simulink model "Feuchtesimulation_G21_EU6AGA_rueckgabewerte"  (R2021b)
settings: Solver=FixedStepAuto  StartTime=start_time  StopTime=stop_time  FixedStep=ts  RelTol=1e-3
undefined symbols (not defined in the file or in its folder): A_Kat0, A_Kat1, A_Kat2, A_Kat3, A_Mantel_Kat0, A_Mantel_Kat1, A_Mantel_Kat2, A_Mantel_Kat3, Air_N2, Air_O2, beladungskennfeld, C_mw, CO2_mw, FeuchteAnsaugluft_rel, FeuchtegradAnsaugluft, Fuel_C, Fuel_H, H2O_mw, H_mw, Kat0_Anzahl_Zonen, Kat1_Anzahl_Zonen, Kat2_Anzahl_Zonen, Kat3_Anzahl_Zonen, l_Kat0, l_Kat1, l_Kat2, l_Kat3, m_Canning_Kat0, m_Canning_Kat1, m_Canning_Kat2, m_Canning_Kat3, m_h2o_kat0_ads, m_h2o_kat0_kond, m_h2o_kat1_ads, m_h2o_kat1_kond, m_h2o_kat2_ads, m_h2o_kat2_kond, m_h2o_kat3_ads, m_h2o_kat3_kond, m_Isolierung_Kat0, m_Isolierung_Kat1, m_Isolierung_Kat2, m_Isolierung_Kat3, m_zeolith_kat0_zone, m_zeolith_kat1_zone, m_zeolith_kat2_zone, m_zeolith_kat3_zone, m_zKat0, m_zKat1, m_zKat2, m_zKat3, Mat_Kat0, Mat_Kat1, Mat_Kat2, Mat_Kat3, N2_mw, O2_mw, p_dsat, Rohr0, Rohr1 ... (+20)
libraries: Feuchtesimulation_Lib x69
(part 3 of 3)

== system Feuchtesimulation_G21_EU6AGA_rueckgabewerte/Rohr nach SCR/T to H ==
  Temperatur [°C] : Inport
  spezifische Feuchte [kg/kg] : Inport  Port=2
  Massenstrom [kg/h] : Inport  Port=3
  Multiply : Product  Inputs=3
  kgph to kgps : Subsystem
  kombinierte Wärmekapazität : Subsystem
  Enthalpiestrom [W] : Outport  VectorParamsAs1DForOutWhenUnconnected=off
  wires:
  Massenstrom [kg/h]/1 -> kgph to kgps/1(kgph)
  Temperatur [°C]/1 -> Multiply/1
  spezifische Feuchte [kg/kg]/1 -> kombinierte Wärmekapazität/1(Spezifische Feuchte)
  Multiply/1 -> Enthalpiestrom [W]/1
  kombinierte Wärmekapazität/1(kombinierte Wärmekapazität) -> Multiply/2
  kgph to kgps/1(kgps) -> Multiply/3

== system Feuchtesimulation_G21_EU6AGA_rueckgabewerte/Rohr nach SCR/kgph to kgps ==
  kgph : Inport
  Constant : Constant  Value=3600
  dm_kgps : Product  Inputs=*/
  kgps : Outport  VectorParamsAs1DForOutWhenUnconnected=off
  wires:
  dm_kgps/1 -> kgps/1
  kgph/1 -> dm_kgps/1
  Constant/1 -> dm_kgps/2

== system Feuchtesimulation_G21_EU6AGA_rueckgabewerte/Rohr vor NSC EXPERIMENTELL/Konfiguration2 ==
  Bus Creator : BusCreator  Inputs=13
  Constant : Constant  Value=Rohr0.Mantelflaeche_innen
  Constant1 : Constant  Value=Rohr0.Mantelflaeche_aussen
  Constant10 : Constant  Value=99
  Constant12 : Constant  Value=Rohr0.Laenge_Abschnitt
  Constant15 : Constant  Value=Rohr0.Waermeleitquerschnitt
  Constant2 : Constant  Value=Rohr0.StroemungsdurchmesserEff
  Constant3 : Constant  Value=Rohr0.thermWidIso
  Constant4 : Constant  Value=Rohr0.Masse_Wasser_start
  Constant5 : Constant  Value=Rohr0.LambdaRohr
  Constant6 : Constant  Value=Rohr0.MasseRohr
  Constant7 : Constant  Value=0
  Constant8 : Constant  Value=Rohr0.Waermekapazitaet
  Constant9 : Constant  Value=Rohr0.thermWidRohr
  From Workspace : FromWorkspace  VariableName=Exh_tAdapTOxiCatUs
  Terminator : Terminator
  Konfiguration : Outport  VectorParamsAs1DForOutWhenUnconnected=off
  wires:
  Bus Creator/1 -> Konfiguration/1
  Constant/1 -> Bus Creator/1  "Mantelfläche innen [m2]"
  Constant1/1 -> Bus Creator/2  "Mantelfläche außen [m2]"
  Constant3/1 -> Bus Creator/4  "r_thermWidIso_m2K/W"
  Constant4/1 -> Bus Creator/5  "Masse Wasser start [kg]"
  Constant12/1 -> Bus Creator/3  "Länge RohrSegment [m]"
  Constant15/1 -> Bus Creator/11  "Wärmeleitquerschnitt Rohr [m2]"
  Constant2/1 -> Bus Creator/7  "gleichwertiger Strömungsdurchmesser [m]"
  Constant5/1 -> Bus Creator/8  "Wärmeleitfähigkeit [W/mK]"
  Constant6/1 -> Bus Creator/9  "Masse Rohr [kg]"
  Constant8/1 -> Bus Creator/10  "Wärmekapazität Rohr [J/kgK]"
  Constant7/1 -> Bus Creator/12  "dummy"
  From Workspace/1 -> Bus Creator/13  "Re-InitialisierungsTemp [degC]"
  Constant9/1 -> Bus Creator/6  "r_thermWidRohr_m2K/W"
  Constant10/1 -> Terminator/1  "Re-InitialisierungsTemp [degC]"

== system Feuchtesimulation_G21_EU6AGA_rueckgabewerte/Rohr vor NSC EXPERIMENTELL/T to H ==
  Temperatur [°C] : Inport
  spezifische Feuchte [kg/kg] : Inport  Port=2
  Massenstrom [kg/h] : Inport  Port=3
  Multiply : Product  Inputs=3
  kgph to kgps : Subsystem
  kombinierte Wärmekapazität : Feuchtesimulation_Lib/Brick/Enthalpiestrom ausgehend /kombinierte Wärmekapazität  SystemSampleTime=-1  VariantActivationTime=update diagram  Latency=0  AutoFrameSizeCalculation=off
  Enthalpiestrom [W] : Outport  VectorParamsAs1DForOutWhenUnconnected=off
  wires:
  Massenstrom [kg/h]/1 -> kgph to kgps/1(kgph)
  Temperatur [°C]/1 -> Multiply/1
  spezifische Feuchte [kg/kg]/1 -> kombinierte Wärmekapazität/1
  Multiply/1 -> Enthalpiestrom [W]/1
  kombinierte Wärmekapazität/1 -> Multiply/2
  kgph to kgps/1(kgps) -> Multiply/3

== system Feuchtesimulation_G21_EU6AGA_rueckgabewerte/Rohr vor NSC EXPERIMENTELL/kgph to kgps ==
  kgph : Inport
  Constant : Constant  Value=3600
  dm_kgps : Product  Inputs=*/
  kgps : Outport  VectorParamsAs1DForOutWhenUnconnected=off
  wires:
  dm_kgps/1 -> kgps/1
  kgph/1 -> dm_kgps/1
  Constant/1 -> dm_kgps/2

== system Feuchtesimulation_G21_EU6AGA_rueckgabewerte/Rohr zwischen DPF und SCR/Konfiguration2 ==
  Bus Creator : BusCreator  Inputs=13
  Constant : Constant  Value=Rohr1.Mantelflaeche_innen
  Constant1 : Constant  Value=Rohr1.Mantelflaeche_aussen
  Constant10 : Constant  Value=99
  Constant12 : Constant  Value=Rohr1.Laenge_Abschnitt
  Constant15 : Constant  Value=Rohr1.Waermeleitquerschnitt
  Constant2 : Constant  Value=Rohr1.StroemungsdurchmesserEff
  Constant3 : Constant  Value=Rohr1.thermWidIso
  Constant4 : Constant  Value=Rohr1.Masse_Wasser_start
  Constant5 : Constant  Value=Rohr1.LambdaRohr
  Constant6 : Constant  Value=Rohr1.MasseRohr
  Constant7 : Constant  Value=0
  Constant8 : Constant  Value=Rohr1.Waermekapazitaet
  Constant9 : Constant  Value=Rohr1.thermWidRohr
  From Workspace : FromWorkspace  VariableName=T_vSCR
  Terminator : Terminator
  Konfiguration : Outport  VectorParamsAs1DForOutWhenUnconnected=off
  wires:
  Bus Creator/1 -> Konfiguration/1
  Constant/1 -> Bus Creator/1  "Mantelfläche innen [m2]"
  Constant1/1 -> Bus Creator/2  "Mantelfläche außen [m2]"
  Constant4/1 -> Bus Creator/5  "Masse Wasser start [kg]"
  Constant12/1 -> Bus Creator/3  "Länge RohrSegment [m]"
  Constant15/1 -> Bus Creator/11  "Wärmeleitquerschnitt Rohr [m2]"
  Constant2/1 -> Bus Creator/7  "gleichwertiger Strömungsdurchmesser [m]"
  Constant5/1 -> Bus Creator/8  "Wärmeleitfähigkeit [W/mK]"
  Constant6/1 -> Bus Creator/9  "Masse Rohr [kg]"
  Constant8/1 -> Bus Creator/10  "Wärmekapazität Rohr [J/kgK]"
  From Workspace/1 -> Bus Creator/13  "Re-InitialisierungsTemp [degC]"
  Constant3/1 -> Bus Creator/4  "r_thermWidIso_m2K/W"
  Constant9/1 -> Bus Creator/6  "r_thermWidRohr_m2K/W"
  Constant7/1 -> Bus Creator/12  "dummy"
  Constant10/1 -> Terminator/1  "Re-InitialisierungsTemp [degC]"

== system Feuchtesimulation_G21_EU6AGA_rueckgabewerte/Rohr zwischen DPF und SCR/T to H ==
  Temperatur [°C] : Inport
  spezifische Feuchte [kg/kg] : Inport  Port=2
  Massenstrom [kg/h] : Inport  Port=3
  Multiply : Product  Inputs=3
  kgph to kgps : Subsystem
  kombinierte Wärmekapazität : Subsystem
  Enthalpiestrom [W] : Outport  VectorParamsAs1DForOutWhenUnconnected=off
  wires:
  Massenstrom [kg/h]/1 -> kgph to kgps/1(kgph)
  Temperatur [°C]/1 -> Multiply/1
  spezifische Feuchte [kg/kg]/1 -> kombinierte Wärmekapazität/1(Spezifische Feuchte)
  Multiply/1 -> Enthalpiestrom [W]/1
  kombinierte Wärmekapazität/1(kombinierte Wärmekapazität) -> Multiply/2
  kgph to kgps/1(kgps) -> Multiply/3

== system Feuchtesimulation_G21_EU6AGA_rueckgabewerte/Rohr zwischen DPF und SCR/kgph to kgps ==
  kgph : Inport
  Constant : Constant  Value=3600
  dm_kgps : Product  Inputs=*/
  kgps : Outport  VectorParamsAs1DForOutWhenUnconnected=off
  wires:
  dm_kgps/1 -> kgps/1
  kgph/1 -> dm_kgps/1
  Constant/1 -> dm_kgps/2

== system Feuchtesimulation_G21_EU6AGA_rueckgabewerte/SCR/Konfig und TInit ==
  ReInitTemp : Inport
  Bus Creator : BusCreator  Inputs=7
  Bus Selector : BusSelector  OutputSignals=Re-InitialisierungsTemp [degC]
  Constant : Constant  Value=RTh_Brick_Iso_Kat2
  Constant1 : Constant  Value=RTh_Iso_Canning_Kat2
  Constant2 : Constant  Value=m_Isolierung_Kat2
  Constant3 : Constant  Value=m_Canning_Kat2
  Constant4 : Constant  Value=A_Mantel_Kat2
  Constant5 : Constant  Value=Kat2_Anzahl_Zonen
  Konfiguration : Outport  VectorParamsAs1DForOutWhenUnconnected=off
  wires:
  Bus Creator/1 -> Konfiguration/1
  Constant/1 -> Bus Creator/1  "RTh_Brick_Iso [K/W]"
  Constant1/1 -> Bus Creator/2  "RTh_Iso_Canning [K/W]"
  Constant3/1 -> Bus Creator/4  "m_Canning [kg]"
  Constant4/1 -> Bus Creator/5  "A_Mantel [m2]"
  Constant5/1 -> Bus Creator/6  "Anzahl_Zonen [-]"
  Constant2/1 -> Bus Creator/3  "m_Isolierung [kg]"
  ReInitTemp/1 -> Bus Selector/1
  Bus Selector/1 -> Bus Creator/7  "<Re-InitialisierungsTemp [degC]>"

== system Feuchtesimulation_G21_EU6AGA_rueckgabewerte/SCR/Konfiguration ==
  Bus Creator : BusCreator  Inputs=10
  Bus Creator1 : BusCreator  Inputs=6
  Constant : Constant  Value=A_Kat2
  Constant1 : Constant  Value=l_Kat2
  Constant10 : Constant  Value=Mat_Kat2.lamda
  Constant11 : Constant  Value=beladungskennfeld.maxAdsBel_prz
  Constant12 : Constant  Value=Kat2_Anzahl_Zonen
  Constant13 : Constant  Value=Mat_Kat2.AeffFaktor
  Constant14 : Constant  Value=99
  Constant2 : Constant  Value=Mat_Kat2.beladung
  Constant3 : Constant  Value=-1
  Constant4 : Constant  Value=m_h2o_kat2_kond
  Constant5 : Constant  Value=m_zeolith_kat2_zone
  Constant6 : Constant  Value=m_h2o_kat2_ads
  Constant7 : Constant  Value=m_zKat2
  Constant8 : Constant  Value=Mat_Kat2.c_c
  Constant9 : Constant  Value=Mat_Kat2.c_T
  From Workspace : FromWorkspace  VariableName=T_nSCR
  Terminator : Terminator
  Konfiguration : Outport  VectorParamsAs1DForOutWhenUnconnected=off
  wires:
  Constant10/1 -> Bus Creator1/5  "Wärmeleitfähigkeit [W/mK]"
  Constant7/1 -> Bus Creator/8  "Masse Bauteil pro Zone [kg]"
  Bus Creator1/1 -> Bus Creator/10  "Material Bauteil"
  Constant1/1 -> Bus Creator/2  "Gesamtlänge Bauteil [m]"
  Constant12/1 -> Bus Creator/3  "Anzahl Zonen [-]"
  Bus Creator/1 -> Konfiguration/1
  Constant9/1 -> Bus Creator1/4  "Wärmekapazität KL Temperatur [°C]"
  Constant8/1 -> Bus Creator1/3  "Wärmekapazität Kennlienie [kJ/kgK]"
  Constant2/1 -> Bus Creator1/2  "Max KondBeladung [kg/kg]"
  Constant5/1 -> Bus Creator/6  "Masse Zeolith pro Zone [kg]"
  Constant4/1 -> Bus Creator/5  "Masse Wasser Kondensation start [kg]"
  Constant6/1 -> Bus Creator/7  "Masse Wasser Adsorption start [kg]"
  Constant/1 -> Bus Creator/1  "Querschnittsfläche Bauteil [m2]"
  Constant13/1 -> Bus Creator1/1  "AeffFaktor [-]"
  Constant11/1 -> Bus Creator1/6  "MaxAdsBelGrad [%]"
  From Workspace/1 -> Bus Creator/9  "Re-InitialisierungsTemp [degC]"
  Constant3/1 -> Bus Creator/4  "dummy"
  Constant14/1 -> Terminator/1  "Re-InitialisierungsTemp [degC]"

== system Feuchtesimulation_G21_EU6AGA_rueckgabewerte/SCR/Subsystem2 ==
  Bel_Ads_% : Inport
  Konfig : Inport  Port=2
  Bus Selector : BusSelector  OutputSignals=Masse Zeolith pro Zone [kg],Material Bauteil.MaxAdsBelGrad [%]
  Gain4 : Gain  Gain=0.1
  Multiply : Product  Inputs=3
  m_H2OAds_g : Outport  VectorParamsAs1DForOutWhenUnconnected=off
  wires:
  Gain4/1 -> m_H2OAds_g/1  "m_Wasser_g"
  Konfig/1 -> Bus Selector/1
  Bel_Ads_%/1 -> Multiply/1
  Bus Selector/2 -> Multiply/3  "<MaxAdsBelGrad [%]>"
  Bus Selector/1 -> Multiply/2  "<Masse Zeolith pro Zone [kg]>"
  Multiply/1 -> Gain4/1  "m*10000_kg"

== system Feuchtesimulation_G21_EU6AGA_rueckgabewerte/SCR/Subsystem3 ==
  Bel_Ads_% : Inport
  Konfig : Inport  Port=2
  Bus Selector : BusSelector  OutputSignals=Masse Zeolith pro Zone [kg],Material Bauteil.MaxAdsBelGrad [%]
  Gain4 : Gain  Gain=0.1
  Multiply : Product  Inputs=3
  m_H2OAds_g : Outport  VectorParamsAs1DForOutWhenUnconnected=off
  wires:
  Gain4/1 -> m_H2OAds_g/1  "m_Wasser_g"
  Konfig/1 -> Bus Selector/1
  Bel_Ads_%/1 -> Multiply/1
  Bus Selector/2 -> Multiply/3  "<MaxAdsBelGrad [%]>"
  Bus Selector/1 -> Multiply/2  "<Masse Zeolith pro Zone [kg]>"
  Multiply/1 -> Gain4/1  "m*10000_kg"

== system Feuchtesimulation_G21_EU6AGA_rueckgabewerte/SCR/kgph to kgps ==
  kgph : Inport
  Constant : Constant  Value=3600
  dm_kgps : Product  Inputs=*/
  kgps : Outport  VectorParamsAs1DForOutWhenUnconnected=off
  wires:
  Constant/1 -> dm_kgps/2
  kgph/1 -> dm_kgps/1
  dm_kgps/1 -> kgps/1

== system Feuchtesimulation_G21_EU6AGA_rueckgabewerte/FeuchteVorgabe/Subsystem1/nantozero1 ==
  input : Inport
  IsNaN : RelationalOperator  Operator=isNaN  OutDataTypeStr=boolean  RndMeth=Simplest
  Switch : Switch  Criteria=u2 > Threshold
  Zero : Constant  OutDataTypeStr=Inherit: Inherit via back propagation
  output : Outport  VectorParamsAs1DForOutWhenUnconnected=off
  wires:
  Switch/1 -> output/1
  IsNaN/1 -> Switch/2
  input/1 -> IsNaN/1, Switch/3
  Zero/1 -> Switch/1

== system Feuchtesimulation_G21_EU6AGA_rueckgabewerte/Rohr nach SCR/T to H/kgph to kgps ==
  kgph : Inport
  Constant : Constant  Value=3600
  dm_kgps : Product  Inputs=*/
  kgps : Outport  VectorParamsAs1DForOutWhenUnconnected=off
  wires:
  dm_kgps/1 -> kgps/1
  kgph/1 -> dm_kgps/1
  Constant/1 -> dm_kgps/2

== system Feuchtesimulation_G21_EU6AGA_rueckgabewerte/Rohr nach SCR/T to H/kombinierte Wärmekapazität ==
  Spezifische Feuchte : Inport
  Constant : Constant
  Constant1 : Constant  Value=waermekapazitaet_wasser_gasfoermig
  Multiply : Product
  Multiply1 : Product
  Sum : Sum  Inputs=|+-
  Sum1 : Sum  Inputs=|++
  cp1 : Constant  Value=waermekapazitaet_luft
  kombinierte Wärmekapazität : Outport  VectorParamsAs1DForOutWhenUnconnected=off
  wires:
  Multiply/1 -> Sum1/2
  Sum/1 -> Multiply/1
  Constant/1 -> Sum/1
  Spezifische Feuchte/1 -> Sum/2, Multiply1/1
  Constant1/1 -> Multiply1/2
  cp1/1 -> Multiply/2
  Multiply1/1 -> Sum1/1
  Sum1/1 -> kombinierte Wärmekapazität/1

== system Feuchtesimulation_G21_EU6AGA_rueckgabewerte/Rohr vor NSC EXPERIMENTELL/T to H/kgph to kgps ==
  kgph : Inport
  Constant : Constant  Value=3600
  dm_kgps : Product  Inputs=*/
  kgps : Outport  VectorParamsAs1DForOutWhenUnconnected=off
  wires:
  dm_kgps/1 -> kgps/1
  kgph/1 -> dm_kgps/1
  Constant/1 -> dm_kgps/2

== system Feuchtesimulation_G21_EU6AGA_rueckgabewerte/Rohr zwischen DPF und SCR/T to H/kgph to kgps ==
  kgph : Inport
  Constant : Constant  Value=3600
  dm_kgps : Product  Inputs=*/
  kgps : Outport  VectorParamsAs1DForOutWhenUnconnected=off
  wires:
  dm_kgps/1 -> kgps/1
  kgph/1 -> dm_kgps/1
  Constant/1 -> dm_kgps/2

== system Feuchtesimulation_G21_EU6AGA_rueckgabewerte/Rohr zwischen DPF und SCR/T to H/kombinierte Wärmekapazität ==
  Spezifische Feuchte : Inport
  Constant : Constant
  Constant1 : Constant  Value=waermekapazitaet_wasser_gasfoermig
  Multiply : Product
  Multiply1 : Product
  Sum : Sum  Inputs=|+-
  Sum1 : Sum  Inputs=|++
  cp1 : Constant  Value=waermekapazitaet_luft
  kombinierte Wärmekapazität : Outport  VectorParamsAs1DForOutWhenUnconnected=off
  wires:
  Multiply/1 -> Sum1/2
  Sum/1 -> Multiply/1
  Constant/1 -> Sum/1
  Spezifische Feuchte/1 -> Sum/2, Multiply1/1
  Constant1/1 -> Multiply1/2
  cp1/1 -> Multiply/2
  Multiply1/1 -> Sum1/1
  Sum1/1 -> kombinierte Wärmekapazität/1

== matlab function Feuchtesimulation_G21_EU6AGA_rueckgabewerte/Relative Feuchte [%]3/Maximale spez Luftf.1 ==
  data: p input; p_dsat input; s_max output
function s_max = fcn(p,p_dsat)
    H2O_mw = 18.02;
    AIR_mw = 28.96;     
s_max = H2O_mw/AIR_mw*p_dsat/(p-(1-H2O_mw/AIR_mw)*p_dsat);

== matlab function Feuchtesimulation_G21_EU6AGA_rueckgabewerte/FeuchteVorgabe/Subsystem2/Mischverhältnis Ansaugluft ==
  data: phi input; x output; p_dsat input; p_0 input
function x = fcn(phi,p_dsat,p_0)

x = (18.01528/28.9644 * p_dsat/(p_0/phi -p_dsat));

== matlab function Feuchtesimulation_G21_EU6AGA_rueckgabewerte/Relative Feuchte [%]1/Maximale spez Luftf.1 ==
  data: p input; p_dsat input; s_max output
function s_max = fcn(p,p_dsat)
    H2O_mw = 18.02;
    AIR_mw = 28.96;     
s_max = H2O_mw/AIR_mw*p_dsat/(p-(1-H2O_mw/AIR_mw)*p_dsat);

== matlab function Feuchtesimulation_G21_EU6AGA_rueckgabewerte/Relative Feuchte [%]2/Maximale spez Luftf.1 ==
  data: p input; p_dsat input; s_max output
function s_max = fcn(p,p_dsat)
    H2O_mw = 18.02;
    AIR_mw = 28.96;     
s_max = H2O_mw/AIR_mw*p_dsat/(p-(1-H2O_mw/AIR_mw)*p_dsat);

== matlab function Feuchtesimulation_G21_EU6AGA_rueckgabewerte/Relative Feuchte [%]4/Maximale spez Luftf.1 ==
  data: p input; p_dsat input; s_max output
function s_max = fcn(p,p_dsat)
    H2O_mw = 18.02;
    AIR_mw = 28.96;     
s_max = H2O_mw/AIR_mw*p_dsat/(p-(1-H2O_mw/AIR_mw)*p_dsat);

== matlab function Feuchtesimulation_G21_EU6AGA_rueckgabewerte/Relative Feuchte [%]5/Maximale spez Luftf.1 ==
  data: p input; p_dsat input; s_max output
function s_max = fcn(p,p_dsat)
    H2O_mw = 18.02;
    AIR_mw = 28.96;     
s_max = H2O_mw/AIR_mw*p_dsat/(p-(1-H2O_mw/AIR_mw)*p_dsat);

== matlab function Feuchtesimulation_G21_EU6AGA_rueckgabewerte/Relative Feuchte [%]6/Maximale spez Luftf.1 ==
  data: p input; p_dsat input; s_max output
function s_max = fcn(p,p_dsat)
    H2O_mw = 18.02;
    AIR_mw = 28.96;     
s_max = H2O_mw/AIR_mw*p_dsat/(p-(1-H2O_mw/AIR_mw)*p_dsat);

== matlab function Feuchtesimulation_G21_EU6AGA_rueckgabewerte/Relative Feuchte [%]/Maximale spez Luftf.1 ==
  data: p input; p_dsat input; s_max output
function s_max = fcn(p,p_dsat)
    H2O_mw = 18.02;
    AIR_mw = 28.96;     
s_max = H2O_mw/AIR_mw*p_dsat/(p-(1-H2O_mw/AIR_mw)*p_dsat);

== matlab function Feuchtesimulation_G21_EU6AGA_rueckgabewerte/FeuchteVorgabe/Subsystem/Mischverhältnis Ansaugluft ==
  data: phi input; x output; p_dsat input; p_0 input
function x = fcn(phi,p_dsat,p_0)

x = (18.01528/28.9644 * p_dsat/(p_0/phi -p_dsat));
